simulink model "progetto_prova_plate"  (R2024a)
settings: Solver=VariableStepAuto  StartTime=0.0  StopTime=20  RelTol=1e-3  AbsTol=1e-3
undefined symbols (not defined in the file or in its folder): X, Y, Z
libraries: sm_lib x23, nesl_utility x10, slpidlib x4
(part 2 of 2)

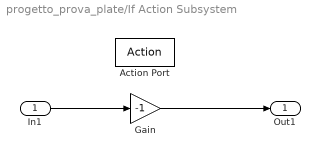
== system progetto_prova_plate/If Action Subsystem ==
  In1 : Inport
  Action Port : ActionPort  ActionPortLabel=else
  Gain : Gain  Gain=-1
  Out1 : Outport
  wires:
  In1/1 -> Gain/1
  Gain/1 -> Out1/1

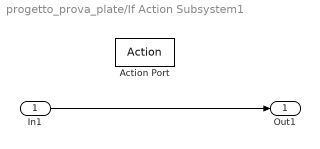
== system progetto_prova_plate/If Action Subsystem1 ==
  In1 : Inport
  Action Port : ActionPort  ActionPortLabel=if(u1 >= 0 )
  Out1 : Outport
  wires:
  In1/1 -> Out1/1

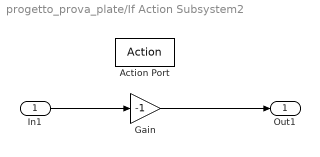
== system progetto_prova_plate/If Action Subsystem2 ==
  In1 : Inport
  Action Port : ActionPort  ActionPortLabel=else
  Gain : Gain  Gain=-1
  Out1 : Outport
  wires:
  In1/1 -> Gain/1
  Gain/1 -> Out1/1

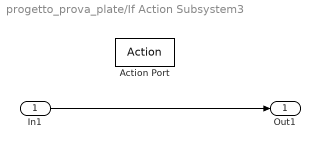
== system progetto_prova_plate/If Action Subsystem3 ==
  In1 : Inport
  Action Port : ActionPort  ActionPortLabel=if(u1 >= 0 )
  Out1 : Outport
  wires:
  In1/1 -> Out1/1

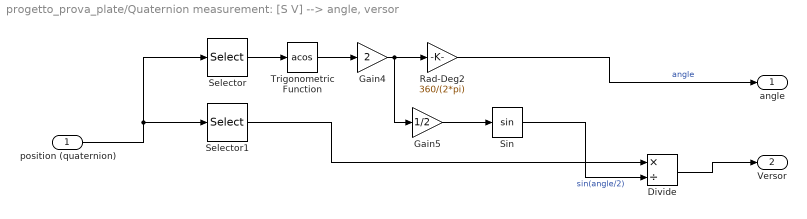
== system progetto_prova_plate/Quaternion measurement: [S V] --> angle, versor ==
  position (quaternion) : Inport
  Divide : Product  Inputs=*/
  Gain4 : Gain  Gain=2
  Gain5 : Gain  Gain=1/2
  Rad-Deg2 : Gain  Gain=360/(2*pi)
  Selector : Selector  InputPortWidth=4  IndexOptions=Index vector (dialog)  Indices=1  OutputSizes=1
  Selector1 : Selector  InputPortWidth=4  IndexOptions=Index vector (dialog)  Indices=2:4  OutputSizes=1
  Sin : Trigonometry
  Trigonometric Function : Trigonometry  Operator=acos
  angle : Outport
  Versor : Outport  Port=2
  wires:
  Gain5/1 -> Sin/1
  Gain4/1 -> Gain5/1, Rad-Deg2/1
  Selector1/1 -> Divide/1
  Trigonometric Function/1 -> Gain4/1
  position (quaternion)/1 -> Selector1/1, Selector/1
  Sin/1 -> Divide/2  "sin(angle/2)"
  Selector/1 -> Trigonometric Function/1
  Divide/1 -> Versor/1
  Rad-Deg2/1 -> angle/1  "angle"
